simulink model "B2B_HVDC_MMC"  (R2023b)
settings: Solver=ode23t  StartTime=0.0  StopTime=3  FixedStep=Ts_Power  MaxStep=1e-3  MinStep=Ts_Power  RelTol=1e-3
values from neighbouring files (symbols this model uses):
  AC_lim = 1*[1.5 -1.5]    [B2B_HVDC_MMC_Calc.m]
  C_pm = 10.48e-3    (= 0.01048)    [B2B_HVDC_MMC_Calc.m]
  Carm = 1.0*C_pm/n    (= 0.0002096)    [B2B_HVDC_MMC_Calc.m]    (also in HVDC_MMC_param.m = 4.88333333333e-05)
  ccsc_lim = 1*[1.0 -1.0]    [B2B_HVDC_MMC_Calc.m]
  DC_lim = 1*[1.05 -1.05]    [B2B_HVDC_MMC_Calc.m]
  f = 50    [B2B_HVDC_MMC_Calc.m]
  Fn_filter = 1000    [B2B_HVDC_MMC_Calc.m]    (also in HVDC_MMC_param.m)
  Fnom = 50    [HVDC_MMC_param.m]
  HrmOrd = N    (= 2)    [B2B_HVDC_MMC_Calc.m]    (also in HVDC_MMC_param.m)
  I_nom = S_nom/(sqrt(3)*V_grid)    [B2B_HVDC_MMC_Calc.m]
  Ireg_lim_i = 1*[1.5, -1.5]    [B2B_HVDC_MMC_Calc.m]
  Ireg_lim_r = 2*[1.5, -1.5]    [B2B_HVDC_MMC_Calc.m]
  Ki_ACreg_i = 260    [B2B_HVDC_MMC_Calc.m]
  Ki_ccsc = 5    [B2B_HVDC_MMC_Calc.m]
  Ki_DCreg_r = 150    [B2B_HVDC_MMC_Calc.m]
  Ki_Ireg_i = 200    [B2B_HVDC_MMC_Calc.m]
  Ki_Ireg_r = 50    [B2B_HVDC_MMC_Calc.m]
  Kp_ACreg_i = 2    [B2B_HVDC_MMC_Calc.m]
  Kp_ccsc = 1    [B2B_HVDC_MMC_Calc.m]
  Kp_DCreg_r = 8    [B2B_HVDC_MMC_Calc.m]
  Kp_Ireg_i = 2    [B2B_HVDC_MMC_Calc.m]
  Kp_Ireg_r = 0.8    [B2B_HVDC_MMC_Calc.m]
  L1_si = L1_pu*Z_base66/w    [B2B_HVDC_MMC_Calc.m]
  L_arm = L_arm_pu*Z_base66/w    [B2B_HVDC_MMC_Calc.m]
  L_arm_pu = 0.15    [B2B_HVDC_MMC_Calc.m]
  N = 2    [B2B_HVDC_MMC_Calc.m]
  P_nom = 220e6    (= 220000000)    [B2B_HVDC_MMC_Calc.m]
  R1_si = R1_pu*Z_base66    [B2B_HVDC_MMC_Calc.m]
  R_arm = 0.03    [B2B_HVDC_MMC_Calc.m]
  R_arm_pu = R_arm/Z_base66    [B2B_HVDC_MMC_Calc.m]
  R_load = 0.6*40    (= 24)    [B2B_HVDC_MMC_Calc.m]
  R_startup = 17    [B2B_HVDC_MMC_Calc.m]    (also in HVDC_MMC_param.m = 400)
  T_fault = 1.4    [B2B_HVDC_MMC_Calc.m]
  Ts = Ts_Power    (= 5e-05)    [B2B_HVDC_MMC_Calc.m]    (also in HVDC_MMC_param.m)
  Ts_Control = Ts_Power    (= 5e-05)    [B2B_HVDC_MMC_Calc.m]    (also in HVDC_MMC_param.m)
  Ts_DQN = MultTs*Ts_Power    (= 5e-05)    [B2B_HVDC_MMC_Calc.m]    (also in HVDC_MMC_param.m)
  Ts_Power = 1*50e-6    (= 5e-05)    [B2B_HVDC_MMC_Calc.m]    (also in HVDC_MMC_param.m)
  V_ac_ref = 1.035    [B2B_HVDC_MMC_Calc.m]
  V_grid = 66e3    (= 66000)    [B2B_HVDC_MMC_Calc.m]
  Vdc_nom = 135e3    (= 135000)    [B2B_HVDC_MMC_Calc.m]
  Vnom_prim = 333e3    (= 333000)    [HVDC_MMC_param.m]
  Xdcpnz = [zeros(6,1), Xpnz]    [B2B_HVDC_MMC_Calc.m]
  Zeta_filter = 1    [B2B_HVDC_MMC_Calc.m]    (also in HVDC_MMC_param.m)
undefined symbols (not defined in the file or in its folder): DiscIntNeverNeededParam, Pcc, Xdcpnz_c
libraries: DQN_Lib x39, simulink x26, eeTransforms x21, spsCurrentMeasurementLib x16, spsHalfBridgeMMCLib x12, spsSeriesRLCBranchLib x12, B2B_HVDC_MMC_Lib x8, spsSecondOrderFilterLib x8, spsAlphaBetaZerotodq0Lib x6, spsabctoAlphaBetaZeroLib x6, spsThreePhaseVIMeasurementLib x4, spsabctodq0Lib x3
(part 1 of 5)
settings Model: NumberOfSteps=1000  SnapshotBufferSize=5000  SnapshotInterval=100  Creator=tslettba  LastModifiedBy=rober
settings SolverCC: ZeroCrossControl=DisableAll  AlgebraicLoopSolver=TrustRegion  InsertRTBMode=Never (minimum delay)  DecoupledContinuousIntegration=on  ODENIntegrationMethod=ode4
settings DataIOCC: InitialState=xFinal  SaveOperatingPoint=on  SaveFormat=Array  SaveOutput=off  SignalLogging=off  DSMLogging=off  SaveTime=off  ReturnWorkspaceOutputs=off
settings OptimizationCC: BooleanDataType=off  EfficientMapNaN2IntZero=off
settings DebuggingCC: ArithmeticOperatorsInVariantConditions=warning
settings HardwareCC: TargetBitPerPointer=64  TargetBitPerSizeT=64  TargetBitPerPtrDiffT=64  TargetLongLongMode=on  TargetIntDivRoundTo=Zero  TargetEndianess=LittleEndian  TargetWordSize=64  TargetHWDeviceType=MATLAB Host  ProdEqTarget=off
settings ModelReferenceCC: EnableRefExpFcnMdlSchedulingChecks=on  ModelReferenceMinAlgLoopOccurrences=on
settings SFSimCC: SimUseLocalCustomCode=off  CustomCodeUndefinedFunction=UseInterfaceOnly
settings RTWCC: RTWUseLocalCustomCode=off  DLArmComputeVersion=19.05
settings CodeAppCC: MaxIdLength=128
settings GRTTargetCC: TargetLangStandard=C89/C90 (ANSI)  CombineOutputUpdateFcns=off  GRTInterface=on
settings SimscapeCC: SimscapeNormalizeSystem=off

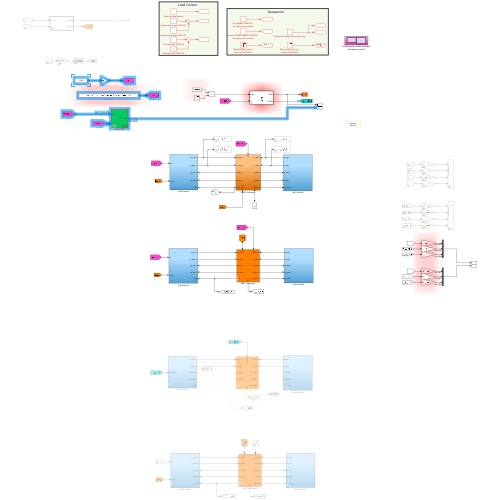
[thumbnail: Simulink's stored preview of the top-level diagram]
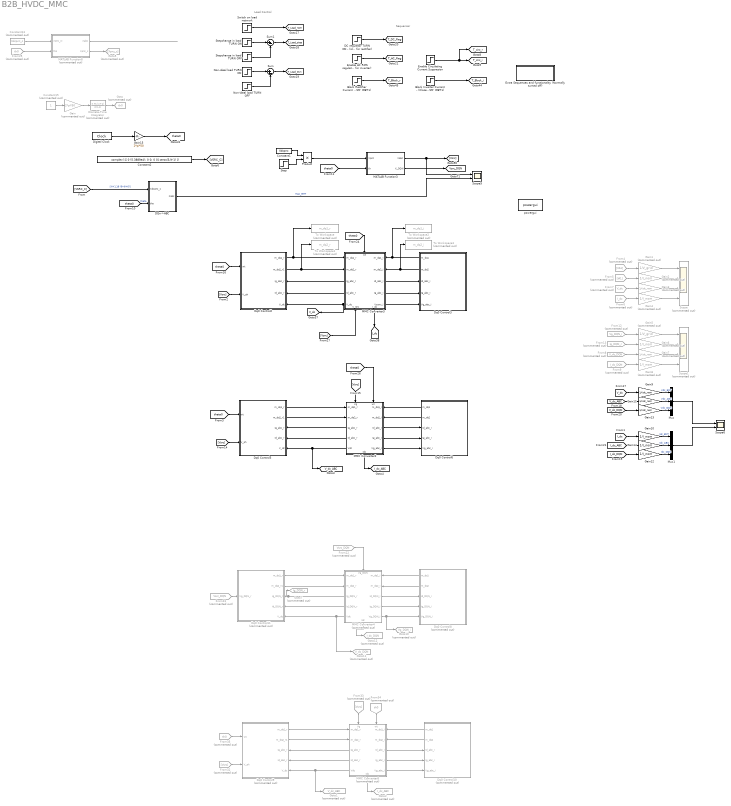
== system B2B_HVDC_MMC ==
  note: Sequencer
  note: Load Control
  Block Inverter Current - (Close all SM' IGBT's) : Step  Time=999999  SampleTime=0
  Block Rectifier Current - (Close all SM' IGBT's) : Step  Time=9999  SampleTime=0
  Constant1 : Constant  Value=Xdcpnz
  Constant13 : Constant  Commented=on  Value=Xdcpnz_c
  Constant15 : Constant  Commented=on
  Constant2 : Constant  Value=complex( [[ 0 (5.3889e4); 0 0; 0 0] zeros(3,N-1) ])
  DC regulator TURN ON - (id reference for rectifier) : Step  Time=0.4  SampleTime=0
  DQn->ABC : MATLAB Function  TreatAsAtomicUnit=on  SystemSampleTime=Ts  mask{N=N}
      mask prompts: N "Harmonic order:"
  Digital Clock : DigitalClock  SampleTime=Ts_Power
  Discrete-Time Integrator : DiscreteIntegrator  Commented=on  IntegratorMethod=Integration: Trapezoidal  SampleTime=Ts_Power  ICPrevOutput=DiscIntNeverNeededParam  ICPrevScaledInput=DiscIntNeverNeededParam
  Dq0 Control10 : Subsystem  Commented=on  VariantControl=Variant1
      settings: PortSchema="{\"entries\":[{\"content\":{\"sides\":[{\"content\":{\"connectorIds\":[]},\"type\":\"ConnectorPlacement.EquallySpacedRectSide\",\"uuid\":\"36f76858-f5b3-4aec-a766-59dc31be5bec\"},{\"content\":{\"connectorIds\":[\"Out1\",\"Out2\",\"In1\",\"In2\",\"In3\"],\"side\":\"RIGHT\"},\"type\":\"ConnectorPlacement.EquallySpacedRectSide\",\"uuid\":\"04787d34-b47d-4ffd-86c1-f3c2e1139151\"},{\"content\":{\"connectorIds\":[],\"side\":\"TOP\"},\"type\":\"ConnectorPlacement.EquallySpacedRectSide\",\"uuid\":\"4aac8492-fb89-4481-9d84-015c15a3650f\"}]},\"type\":\"ConnectorPlacement.EquallySpacedConnector\",\"uuid\":\"f0857c10-9101-4944-b9c2-34b9561f63da\"}],\"packageUris\":[\"http://schema.mathworks.com/mf0/Connector/R2020b\"],\"version\":\"1.0\"}"
  Dq0 Control11 : Subsystem  Commented=on  VariantControl=Variant1
      settings: PortSchema="{\"entries\":[{\"content\":{\"sides\":[{\"content\":{\"connectorIds\":[\"In1\"]},\"type\":\"ConnectorPlacement.EquallySpacedRectSide\",\"uuid\":\"5054124d-5268-420b-bfb4-2e4b28f216ef\"},{\"content\":{\"connectorIds\":[\"Out1\",\"Out2\",\"In2\",\"In3\",\"In4\"],\"side\":\"RIGHT\"},\"type\":\"ConnectorPlacement.EquallySpacedRectSide\",\"uuid\":\"36fdee57-87fd-4c50-8645-9d62359766d9\"},{\"content\":{\"connectorIds\":[],\"side\":\"TOP\"},\"type\":\"ConnectorPlacement.EquallySpacedRectSide\",\"uuid\":\"7247bb4b-18a5-4014-81f5-18aef71126d1\"}]},\"type\":\"ConnectorPlacement.EquallySpacedConnector\",\"uuid\":\"c58730e1-91aa-4896-a8ed-35fe7a3c59a5\"}],\"packageUris\":[\"http://schema.mathworks.com/mf0/Connector/R2020b\"],\"version\":\"1.0\"}"
  Dq0 Control2 : Subsystem  VariantControl=Variant1
      settings: PortSchema="{\"entries\":[{\"content\":{\"sides\":[{\"content\":{\"connectorIds\":[\"In1\",\"In2\"]},\"type\":\"ConnectorPlacement.EquallySpacedRectSide\",\"uuid\":\"5054124d-5268-420b-bfb4-2e4b28f216ef\"},{\"content\":{\"connectorIds\":[\"Out1\",\"Out2\",\"In3\",\"In4\",\"In5\"],\"side\":\"RIGHT\"},\"type\":\"ConnectorPlacement.EquallySpacedRectSide\",\"uuid\":\"36fdee57-87fd-4c50-8645-9d62359766d9\"},{\"content\":{\"connectorIds\":[],\"side\":\"TOP\"},\"type\":\"ConnectorPlacement.EquallySpacedRectSide\",\"uuid\":\"7247bb4b-18a5-4014-81f5-18aef71126d1\"}]},\"type\":\"ConnectorPlacement.EquallySpacedConnector\",\"uuid\":\"c58730e1-91aa-4896-a8ed-35fe7a3c59a5\"}],\"packageUris\":[\"http://schema.mathworks.com/mf0/Connector/R2020b\"],\"version\":\"1.0\"}"
  Dq0 Control3 : Subsystem  VariantControl=Variant1
      settings: PortSchema="{\"entries\":[{\"content\":{\"sides\":[{\"content\":{\"connectorIds\":[]},\"type\":\"ConnectorPlacement.EquallySpacedRectSide\",\"uuid\":\"36f76858-f5b3-4aec-a766-59dc31be5bec\"},{\"content\":{\"connectorIds\":[\"Out1\",\"Out2\",\"In1\",\"In2\",\"In3\"],\"side\":\"RIGHT\"},\"type\":\"ConnectorPlacement.EquallySpacedRectSide\",\"uuid\":\"04787d34-b47d-4ffd-86c1-f3c2e1139151\"},{\"content\":{\"connectorIds\":[],\"side\":\"TOP\"},\"type\":\"ConnectorPlacement.EquallySpacedRectSide\",\"uuid\":\"4aac8492-fb89-4481-9d84-015c15a3650f\"}]},\"type\":\"ConnectorPlacement.EquallySpacedConnector\",\"uuid\":\"f0857c10-9101-4944-b9c2-34b9561f63da\"}],\"packageUris\":[\"http://schema.mathworks.com/mf0/Connector/R2020b\"],\"version\":\"1.0\"}"
  Dq0 Control5 : Subsystem  VariantControl=Variant1
      settings: PortSchema="{\"entries\":[{\"content\":{\"sides\":[{\"content\":{\"connectorIds\":[\"In1\",\"In2\"]},\"type\":\"ConnectorPlacement.EquallySpacedRectSide\",\"uuid\":\"5054124d-5268-420b-bfb4-2e4b28f216ef\"},{\"content\":{\"connectorIds\":[\"Out1\",\"Out2\",\"In3\",\"In4\",\"In5\"],\"side\":\"RIGHT\"},\"type\":\"ConnectorPlacement.EquallySpacedRectSide\",\"uuid\":\"36fdee57-87fd-4c50-8645-9d62359766d9\"},{\"content\":{\"connectorIds\":[],\"side\":\"TOP\"},\"type\":\"ConnectorPlacement.EquallySpacedRectSide\",\"uuid\":\"7247bb4b-18a5-4014-81f5-18aef71126d1\"}]},\"type\":\"ConnectorPlacement.EquallySpacedConnector\",\"uuid\":\"c58730e1-91aa-4896-a8ed-35fe7a3c59a5\"}],\"packageUris\":[\"http://schema.mathworks.com/mf0/Connector/R2020b\"],\"version\":\"1.0\"}"
  Dq0 Control6 : Subsystem  VariantControl=Variant1
      settings: PortSchema="{\"entries\":[{\"content\":{\"sides\":[{\"content\":{\"connectorIds\":[]},\"type\":\"ConnectorPlacement.EquallySpacedRectSide\",\"uuid\":\"36f76858-f5b3-4aec-a766-59dc31be5bec\"},{\"content\":{\"connectorIds\":[\"Out1\",\"Out2\",\"In1\",\"In2\",\"In3\"],\"side\":\"RIGHT\"},\"type\":\"ConnectorPlacement.EquallySpacedRectSide\",\"uuid\":\"04787d34-b47d-4ffd-86c1-f3c2e1139151\"},{\"content\":{\"connectorIds\":[],\"side\":\"TOP\"},\"type\":\"ConnectorPlacement.EquallySpacedRectSide\",\"uuid\":\"4aac8492-fb89-4481-9d84-015c15a3650f\"}]},\"type\":\"ConnectorPlacement.EquallySpacedConnector\",\"uuid\":\"f0857c10-9101-4944-b9c2-34b9561f63da\"}],\"packageUris\":[\"http://schema.mathworks.com/mf0/Connector/R2020b\"],\"version\":\"1.0\"}"
  Dq0 Control8 : Subsystem  Commented=on  VariantControl=Variant1
      settings: PortSchema="{\"entries\":[{\"content\":{\"sides\":[{\"content\":{\"connectorIds\":[]},\"type\":\"ConnectorPlacement.EquallySpacedRectSide\",\"uuid\":\"36f76858-f5b3-4aec-a766-59dc31be5bec\"},{\"content\":{\"connectorIds\":[\"Out1\",\"Out2\",\"In1\",\"In2\",\"In3\"],\"side\":\"RIGHT\"},\"type\":\"ConnectorPlacement.EquallySpacedRectSide\",\"uuid\":\"04787d34-b47d-4ffd-86c1-f3c2e1139151\"},{\"content\":{\"connectorIds\":[],\"side\":\"TOP\"},\"type\":\"ConnectorPlacement.EquallySpacedRectSide\",\"uuid\":\"4aac8492-fb89-4481-9d84-015c15a3650f\"}]},\"type\":\"ConnectorPlacement.EquallySpacedConnector\",\"uuid\":\"f0857c10-9101-4944-b9c2-34b9561f63da\"}],\"packageUris\":[\"http://schema.mathworks.com/mf0/Connector/R2020b\"],\"version\":\"1.0\"}"
  Dq0 Control9 : Subsystem  Commented=on  VariantControl=Variant1
      settings: PortSchema="{\"entries\":[{\"content\":{\"sides\":[{\"content\":{\"connectorIds\":[\"In1\",\"In2\"]},\"type\":\"ConnectorPlacement.EquallySpacedRectSide\",\"uuid\":\"5054124d-5268-420b-bfb4-2e4b28f216ef\"},{\"content\":{\"connectorIds\":[\"Out1\",\"Out2\",\"In3\",\"In4\",\"In5\"],\"side\":\"RIGHT\"},\"type\":\"ConnectorPlacement.EquallySpacedRectSide\",\"uuid\":\"36fdee57-87fd-4c50-8645-9d62359766d9\"},{\"content\":{\"connectorIds\":[],\"side\":\"TOP\"},\"type\":\"ConnectorPlacement.EquallySpacedRectSide\",\"uuid\":\"7247bb4b-18a5-4014-81f5-18aef71126d1\"}]},\"type\":\"ConnectorPlacement.EquallySpacedConnector\",\"uuid\":\"c58730e1-91aa-4896-a8ed-35fe7a3c59a5\"}],\"packageUris\":[\"http://schema.mathworks.com/mf0/Connector/R2020b\"],\"version\":\"1.0\"}"
  Enable AC RMS regulator TURN ON - (id reference for inverter) : Step  Time=0.5  SampleTime=0  ZeroCross=off
  Enable Circulating Current Suppresion : Step  SampleTime=0
  Extra Sequences and functionality (Normally turned off) : Subsystem
  From12 : From  Commented=on  GotoTag=Vg_DQN_i  TagVisibility=global
  From13 : From  Commented=on  GotoTag=Ig_DQN_r  TagVisibility=global
  From22 : From  Commented=on  GotoTag=Vsrc_DQN  TagVisibility=global
  From23 : From  Commented=on  GotoTag=Vsrc_DQN  TagVisibility=global
  From25 : From  Commented=on  GotoTag=th0  TagVisibility=global
  From32 : From  Commented=on  GotoTag=Vsrc
  From33 : From  Commented=on  GotoTag=Vsrc
  From34 : From  Commented=on  GotoTag=th0  TagVisibility=global
  From35 : From  Commented=on  GotoTag=th0  TagVisibility=global
  From4 : From  Commented=on  GotoTag=VA1  TagVisibility=global
  From5 : From  Commented=on  GotoTag=IA1  TagVisibility=global
  From6 : From  Commented=on  GotoTag=I_dc  TagVisibility=global
  From7 : From  Commented=on  GotoTag=V_dc  TagVisibility=global
  From8 : From  Commented=on  GotoTag=V_dc_DQN  TagVisibility=global
  From9 : From  Commented=on  GotoTag=I_dc_DQN  TagVisibility=global
  Gain : Gain  Commented=on  Gain=2*pi*50
  Gain1 : Gain  Commented=on  Gain=1/V_grid
  Gain10 : Gain  Gain=1/I_nom
  Gain11 : Gain  Gain=1/Vdc_nom
  Gain12 : Gain  Gain=1/I_nom
  Gain13 : Gain  Gain=1/Vdc_nom
  Gain14 : Gain  Gain=1/I_nom
  Gain15 : Gain  Gain=2*pi*50
  Gain{2,4,6,8} (4 alike) : Gain  Commented=on  Gain=1/I_nom
  Gain3 : Gain  Commented=on  Gain=1/Vdc_nom
  Gain5 : Gain  Commented=on  Gain=1/V_grid
  Gain7 : Gain  Commented=on  Gain=1/Vdc_nom
  Gain9 : Gain  Gain=1/Vdc_nom
  Goto : Goto  Commented=on  GotoTag=th0  TagVisibility=global
  Goto1 : Goto  Commented=on  GotoTag=V_dc_ABC  TagVisibility=global
  Goto10 : Goto  Commented=on  GotoTag=Vg_DQN_i  TagVisibility=global
  Goto11 : Goto  Commented=on  GotoTag=V_dc_DQN  TagVisibility=global
  Goto12 : Goto  Commented=on  GotoTag=I_dc_DQN  TagVisibility=global
  Goto2 : Goto  Commented=on  GotoTag=I_dc_ABC  TagVisibility=global
  Goto5 : Goto  Commented=on  GotoTag=Xpnz_c
  Goto7 : Goto  Commented=on  GotoTag=Ig_DQN_r  TagVisibility=global
  MATLAB Function3 : MATLAB Function  TreatAsAtomicUnit=on  mask{chkHrmLst=off, HRM=N, HrmLst=[0 7 8]}
      mask prompts: chkHrmLst "Only specific harmonics"; HRM "Harmonic order:"; HrmLst "Harmonic list:"
  MATLAB Function8 : MATLAB Function  Commented=on  TreatAsAtomicUnit=on  mask{chkHrmLst=off, HRM=N, HrmLst=[0 7 8]}
      mask prompts: chkHrmLst "Only specific harmonics"; HRM "Harmonic order:"; HrmLst "Harmonic list:"
  MMC Converter2 : Subsystem  mask{Ts_Power=Ts_DQN}
      mask prompts: Ts_Power "Sample time:"
      settings: PortSchema="{\"entries\":[{\"content\":{\"sides\":[{\"content\":{\"connectorIds\":[\"In1\",\"In2\",\"Out5\",\"Out6\",\"Out7\"]},\"type\":\"ConnectorPlacement.EquallySpacedRectSide\",\"uuid\":\"87652525-d4f3-48bd-afb9-55813d4b97b9\"},{\"content\":{\"connectorIds\":[\"In5\",\"In6\",\"Out1\",\"Out2\",\"Out3\"],\"side\":\"RIGHT\"},\"type\":\"ConnectorPlacement.EquallySpacedRectSide\",\"uuid\":\"55382f73-b2a1-4e3c-9356-c55b2c306da5\"},{\"content\":{\"connectorIds\":[\"In3\",\"In4\"],\"side\":\"TOP\"},\"type\":\"ConnectorPlacement.EquallySpacedRectSide\",\"uuid\":\"5746e390-86c5-411c-b1f1-99edaaeabbe1\"},{\"content\":{\"connectorIds\":[\"Out4\"],\"side\":\"BOTTOM\"},\"type\":\"ConnectorPlacement.EquallySpacedRectSide\",\"uuid\":\"499a406e-551e-409c-998b-1d8f3bc160f4\"}]},\"type\":\"ConnectorPlacement.EquallySpacedConnector\",\"uuid\":\"6141d85e-66b3-4906-aa89-7ac82b0805e9\"}],\"packageUris\":[\"http://schema.mathworks.com/mf0/Connector/R2020b\"],\"version\":\"1.0\"}"
  MMC Converter3 : Subsystem
      settings: PortSchema="{\"entries\":[{\"content\":{\"sides\":[{\"content\":{\"connectorIds\":[\"In1\",\"In2\",\"Out5\",\"Out6\",\"Out7\"]},\"type\":\"ConnectorPlacement.EquallySpacedRectSide\",\"uuid\":\"87652525-d4f3-48bd-afb9-55813d4b97b9\"},{\"content\":{\"connectorIds\":[\"In5\",\"In6\",\"Out1\",\"Out2\",\"Out3\"],\"side\":\"RIGHT\"},\"type\":\"ConnectorPlacement.EquallySpacedRectSide\",\"uuid\":\"55382f73-b2a1-4e3c-9356-c55b2c306da5\"},{\"content\":{\"connectorIds\":[\"In3\"],\"side\":\"TOP\"},\"type\":\"ConnectorPlacement.EquallySpacedRectSide\",\"uuid\":\"5746e390-86c5-411c-b1f1-99edaaeabbe1\"},{\"content\":{\"connectorIds\":[\"In4\",\"Out4\"],\"side\":\"BOTTOM\"},\"type\":\"ConnectorPlacement.EquallySpacedRectSide\",\"uuid\":\"499a406e-551e-409c-998b-1d8f3bc160f4\"}]},\"type\":\"ConnectorPlacement.EquallySpacedConnector\",\"uuid\":\"6141d85e-66b3-4906-aa89-7ac82b0805e9\"}],\"packageUris\":[\"http://schema.mathworks.com/mf0/Connector/R2020b\"],\"version\":\"1.0\"}"
  MMC Converter4 : Subsystem  Commented=on  mask{Ts_Power=Ts_DQN}
      mask prompts: Ts_Power "Sample time (s):"
      settings: PortSchema="{\"entries\":[{\"content\":{\"sides\":[{\"content\":{\"connectorIds\":[\"In1\",\"In2\",\"Out5\",\"Out6\",\"Out7\"]},\"type\":\"ConnectorPlacement.EquallySpacedRectSide\",\"uuid\":\"87652525-d4f3-48bd-afb9-55813d4b97b9\"},{\"content\":{\"connectorIds\":[\"In4\",\"In5\",\"Out1\",\"Out2\",\"Out3\"],\"side\":\"RIGHT\"},\"type\":\"ConnectorPlacement.EquallySpacedRectSide\",\"uuid\":\"55382f73-b2a1-4e3c-9356-c55b2c306da5\"},{\"content\":{\"connectorIds\":[\"In3\"],\"side\":\"TOP\"},\"type\":\"ConnectorPlacement.EquallySpacedRectSide\",\"uuid\":\"5746e390-86c5-411c-b1f1-99edaaeabbe1\"},{\"content\":{\"connectorIds\":[\"Out4\"],\"side\":\"BOTTOM\"},\"type\":\"ConnectorPlacement.EquallySpacedRectSide\",\"uuid\":\"499a406e-551e-409c-998b-1d8f3bc160f4\"}]},\"type\":\"ConnectorPlacement.EquallySpacedConnector\",\"uuid\":\"6141d85e-66b3-4906-aa89-7ac82b0805e9\"}],\"packageUris\":[\"http://schema.mathworks.com/mf0/Connector/R2020b\"],\"version\":\"1.0\"}"
  MMC Converter8 : Subsystem  Commented=on  mask{Ts_Power=Ts_DQN}
      mask prompts: Ts_Power "Sample time:"
      settings: PortSchema="{\"entries\":[{\"content\":{\"sides\":[{\"content\":{\"connectorIds\":[\"In1\",\"In2\",\"Out5\",\"Out6\",\"Out7\"]},\"type\":\"ConnectorPlacement.EquallySpacedRectSide\",\"uuid\":\"87652525-d4f3-48bd-afb9-55813d4b97b9\"},{\"content\":{\"connectorIds\":[\"In5\",\"In6\",\"Out1\",\"Out2\",\"Out3\"],\"side\":\"RIGHT\"},\"type\":\"ConnectorPlacement.EquallySpacedRectSide\",\"uuid\":\"55382f73-b2a1-4e3c-9356-c55b2c306da5\"},{\"content\":{\"connectorIds\":[\"In3\",\"In4\"],\"side\":\"TOP\"},\"type\":\"ConnectorPlacement.EquallySpacedRectSide\",\"uuid\":\"5746e390-86c5-411c-b1f1-99edaaeabbe1\"},{\"content\":{\"connectorIds\":[\"Out4\"],\"side\":\"BOTTOM\"},\"type\":\"ConnectorPlacement.EquallySpacedRectSide\",\"uuid\":\"499a406e-551e-409c-998b-1d8f3bc160f4\"}]},\"type\":\"ConnectorPlacement.EquallySpacedConnector\",\"uuid\":\"6141d85e-66b3-4906-aa89-7ac82b0805e9\"}],\"packageUris\":[\"http://schema.mathworks.com/mf0/Connector/R2020b\"],\"version\":\"1.0\"}"
  Mux : Mux  Inputs=3
  Mux1 : Mux  Inputs=3
  Non-ideal load TURN OFF : Step  Time=2.2*999  SampleTime=0
  Non-ideal load TURN ON : Step  Time=0.7  SampleTime=0
  Product : Product
  Scope : Scope  Commented=on  NumInputPorts=4
  Scope1 : Scope  Commented=on  NumInputPorts=4
  Scope5 : Scope  NumInputPorts=2
  Scope6 : Scope  NumInputPorts=2
  Step : Step  Time=2  Before=1  After=1.15  SampleTime=0
  Stepchange in load TURN OFF : Step  Time=999  SampleTime=0
  Stepchange in load TURN ON : Step  Time=2*9999999  SampleTime=0
  Sum : Sum  Inputs=|+-
  Sum1 : Sum  Inputs=|+-
  Switch on load network : Step  Time=0.3+0*0.6  SampleTime=0
  To Workspace : ToWorkspace  Commented=on  VariableName=m_dq1_r  SaveFormat=Timeseries  SampleTime=Ts_Power
      settings: MaxDataPoints=1
  To Workspace1 : ToWorkspace  Commented=on  VariableName=m_dq2_r  SaveFormat=Timeseries  SampleTime=Ts_Power
      settings: MaxDataPoints=1
  To Workspace2 : ToWorkspace  Commented=on  VariableName=m_dq1_i  SaveFormat=Timeseries  SampleTime=Ts_Power
      settings: MaxDataPoints=1
  To Workspace3 : ToWorkspace  Commented=on  VariableName=m_dq2_i  SaveFormat=Timeseries  SampleTime=Ts_Power
      settings: MaxDataPoints=1
  powergui : spspowerguiLib/powergui  Priority=1  SimulationMode=Discrete  SampleTime=Ts_Power  frequency=60  Iterations=50  frequencyindice=50  Pbase=100e6  ErrMax=1e-4  UnitsV=kV  UnitsW=MW  buscounter=0  FunctionMessages=off  echomessages=off  EnableUseOfTLC=off  CurrentSourceSwitches=off  DisableSnubberDevices=off  DisableRonSwitches=off  DisableVfSwitches=off  DisplayEquations=off  AutomaticDiscreteSolvers=on  SolverType=Tustin/Backward Euler (TBE)  Interpol=off  ExternalGateDelay=off  methode=off  Ts=100  x0status=blocks  SPID=on  SwTol=0  HookPort=off  NonlinearTolerance=1e-4  nMaxIteration=100  ContinueOnMaxIteration=off  RestoreLinks=warning  ResistiveCurrentMeasurement=off  Frange=[0:10:1000000]  Ylog=off  Xlog=on  ShowGrid=on  save=off  variable=ZData  structure=I_inv  ZoomFFT=off  StartTime=2  cycles=1  DisplayStyle=1  fundamental=50  FreqAxis=on  MaxFrequency=3000  frequencyindicesteady=1  RmsSteady=1  display=off
  tag scope: I_dc=global, I_dc_ABC=global, T_AC_Reg=global, T_Block_i=global, T_Block_r=global, T_DC_Reg=global, T_Load_Dyn=global, T_Load_nom=global, T_Load_step=global, T_circ_i=global, T_circ_r=global, V_dc=global, V_dc_ABC=global, Vsrc_DQN=global, theta0=global
  wires:
  Non-ideal load TURN ON/1 -> Sum/1
  Non-ideal load TURN OFF/1 -> Sum/2
  Switch on load network/1 -> [T_Load_nom]
  Sum/1 -> [T_Load_Dyn]
  Stepchange in load TURN OFF/1 -> Sum1/2
  Stepchange in load TURN ON/1 -> Sum1/1
  Sum1/1 -> [T_Load_step]
  DC regulator TURN ON - (id reference for rectifier)/1 -> [T_DC_Reg]
  Enable AC RMS regulator TURN ON - (id reference for inverter)/1 -> [T_AC_Reg]
  Enable Circulating Current Suppresion/1 -> [T_circ_r], [T_circ_i]
  Block Inverter Current - (Close all SM' IGBT's)/1 -> [T_Block_i]
  Block Rectifier Current - (Close all SM' IGBT's)/1 -> [T_Block_r]
  Constant15/1 -> Gain/1
  Discrete-Time Integrator/1 -> Goto/1
  Gain/1 -> Discrete-Time Integrator/1
  MMC Converter3/2(Ig_abc_i) -> Dq0 Control3/2(Ig_abc_i)
  Dq0 Control2/2(m_dq2_r1) -> To Workspace1/1, MMC Converter3/2(m_dq2_r)
  Dq0 Control3/1(m_dq1) -> To Workspace2/1, MMC Converter3/5(m_dq1_i)
  MMC Converter3/6(Id_abc_r) -> Dq0 Control2/4(Id_abc_r)
  MMC Converter3/7(V_dc) -> Dq0 Control2/5(V_dc), [V_dc]
  MMC Converter3/1(Id_abc_i) -> Dq0 Control3/1(Id_abc_i)
  Dq0 Control3/2(m_dq2) -> To Workspace3/1, MMC Converter3/6(m_dq2_i)
  [theta0] -> MMC Converter3/3(wt)
  MMC Converter3/3(Vconv_i) -> Dq0 Control3/3(Vg_abc_i)
  Dq0 Control2/1(m_dq1_r) -> To Workspace/1, MMC Converter3/1(m_dq1_r)
  MMC Converter3/4(I_dc) -> [I_dc]
  [Vsrc] -> Dq0 Control2/2(V_ph)
  [theta0] -> Dq0 Control2/1(wt)
  MMC Converter3/5(Ig_abc_r) -> Dq0 Control2/3(Ig_abc_r)
  Constant1/1 -> Product/1
  Step/1 -> Product/2
  MATLAB Function3/2(X_DQN) -> [Vsrc_DQN]
  MATLAB Function3/1(Xabc) -> Scope5/1, [Vsrc]
  [theta0] -> MATLAB Function3/2(th)
  Product/1 -> MATLAB Function3/1(Xpnz)
  Gain1/1 -> Scope/1
  Gain2/1 -> Scope/2
  Gain3/1 -> Scope/3
  Gain4/1 -> Scope/4
  Gain7/1 -> Scope1/3
  Gain8/1 -> Scope1/4
  From9/1 -> Gain8/1
  From8/1 -> Gain7/1
  Gain6/1 -> Scope1/2
  From12/1 -> Gain5/1
  Gain5/1 -> Scope1/1
  From13/1 -> Gain6/1
  From5/1 -> Gain2/1
  From7/1 -> Gain3/1
  From4/1 -> Gain1/1
  From6/1 -> Gain4/1
  [Vsrc] -> MMC Converter3/4(V_Src)
  MMC Converter2/2(Ig_abc_i) -> Dq0 Control6/2(Ig_abc_i)
  [Vsrc] -> Dq0 Control5/2(V_ph)
  [theta0] -> MMC Converter2/4(wt)
  MMC Converter2/5(Ig_abc_r) -> Dq0 Control5/3(Ig_abc_r)
  [Vsrc] -> MMC Converter2/3(Vg)
  MMC Converter2/3(Vg_abc_i) -> Dq0 Control6/3(Vg_abc_i)
  MMC Converter2/1(Id_abc_i) -> Dq0 Control6/1(Id_abc_i)
  MMC Converter2/6(Id_abc_r) -> Dq0 Control5/4(Id_abc_r)
  [theta0] -> Dq0 Control5/1(wt)
  Mux1/1 -> Scope6/2
  Mux/1 -> Scope6/1
  [I_dc] -> Gain10/1
  [I_dc_DQN] -> Gain12/1
  Gain11/1 -> Mux/2  "Vdc_ABC"
  [V_dc_DQN] -> Gain13/1
  Gain13/1 -> Mux/3  "Vdc_DQN"
  [V_dc] -> Gain9/1
  [V_dc_ABC] -> Gain11/1
  Gain9/1 -> Mux/1  "Vdc_EMT"
  Gain10/1 -> Mux1/1  "Idc_EMT"
  Gain12/1 -> Mux1/3  "Idc_DQN"
  [I_dc_ABC] -> Gain14/1
  Gain14/1 -> Mux1/2  "Idc_ABC"
  Dq0 Control11/2(m_dq2_r1) -> MMC Converter4/2(m_dq2_r)
  From22/1 -> MMC Converter4/3(Vg_DQN)
  Dq0 Control8/1(m_dq1) -> MMC Converter4/4(m_dq1_i)
  Dq0 Control11/1(m_dq1_r) -> MMC Converter4/1(m_dq1_r)
  Dq0 Control8/2(m_dq2) -> MMC Converter4/5(m_dq2_i)
  From23/1 -> Dq0 Control11/1(Vg_DQN_r)
  MMC Converter4/4(Idc) -> Goto12/1
  MMC Converter4/5(Ig_DQN_r) -> Goto7/1, Dq0 Control11/2(Ig_DQN_r)
  MMC Converter4/6(Id_DQN_r) -> Dq0 Control11/3(Id_DQN_r)
  MMC Converter4/1(Id_DQN_i) -> Dq0 Control8/1(Id_DQN_i)
  MMC Converter4/2(Ig_DQN_i) -> Dq0 Control8/2(Ig_DQN_i)
  MMC Converter4/3(Vg_DQN_i) -> Dq0 Control8/3(Vg_DQN_i), Goto10/1
  Dq0 Control5/1(m_dq1_r) -> MMC Converter2/1(m_dq1_r)
  Dq0 Control5/2(m_dq2_r1) -> MMC Converter2/2(m_dq2_r)
  Dq0 Control6/1(m_dq1) -> MMC Converter2/5(m_dq1_i)
  Dq0 Control6/2(m_dq2) -> MMC Converter2/6(m_dq2_i)
  MMC Converter8/3(Vg_abc_i) -> Dq0 Control10/3(Vg_abc_i)
  MMC Converter8/5(Ig_abc_r) -> Dq0 Control9/3(Ig_abc_r)
  MMC Converter8/6(Id_abc_r) -> Dq0 Control9/4(Id_abc_r)
  MMC Converter8/1(Id_abc_i) -> Dq0 Control10/1(Id_abc_i)
  From34/1 -> MMC Converter8/4(wt)
  From32/1 -> Dq0 Control9/2(V_ph)
  MMC Converter8/7(Vdc) -> Dq0 Control9/5(V_dc), Goto1/1
  From35/1 -> Dq0 Control9/1(wt)
  From33/1 -> MMC Converter8/3(Vg)
  Dq0 Control10/2(m_dq2) -> MMC Converter8/6(m_dq2_i)
  MMC Converter8/4(Idc) -> Goto2/1
  Dq0 Control10/1(m_dq1) -> MMC Converter8/5(m_dq1_i)
  Dq0 Control9/1(m_dq1_r) -> MMC Converter8/1(m_dq1_r)
  MMC Converter8/2(Ig_abc_i) -> Dq0 Control10/2(Ig_abc_i)
  Dq0 Control9/2(m_dq2_r1) -> MMC Converter8/2(m_dq2_r)
  MMC Converter2/4(Idc) -> [I_dc_ABC]
  MMC Converter2/7(Vdc) -> [V_dc_ABC], Dq0 Control5/5(V_dc)
  MMC Converter4/7(Vdc) -> Dq0 Control11/4(V_dc), Goto11/1
  Gain15/1 -> [theta0]
  Digital Clock/1 -> Gain15/1
  From25/1 -> MATLAB Function8/2(tho)
  MATLAB Function8/1(Xabc) -> ?
  MATLAB Function8/2(Xpnz_c) -> Goto5/1
  Constant13/1 -> MATLAB Function8/1(Xpnz_ci)
  Constant2/1 -> [VSRC_C]
  [theta0] -> DQn->ABC/2(tho)  "theta"
  [VSRC_C] -> DQn->ABC/1(Xdcpnz_c)  "[N+1,18 (6+6+6)]"
  DQn->ABC/1(Xabc) -> Scope5/2  "Mac_EMT"

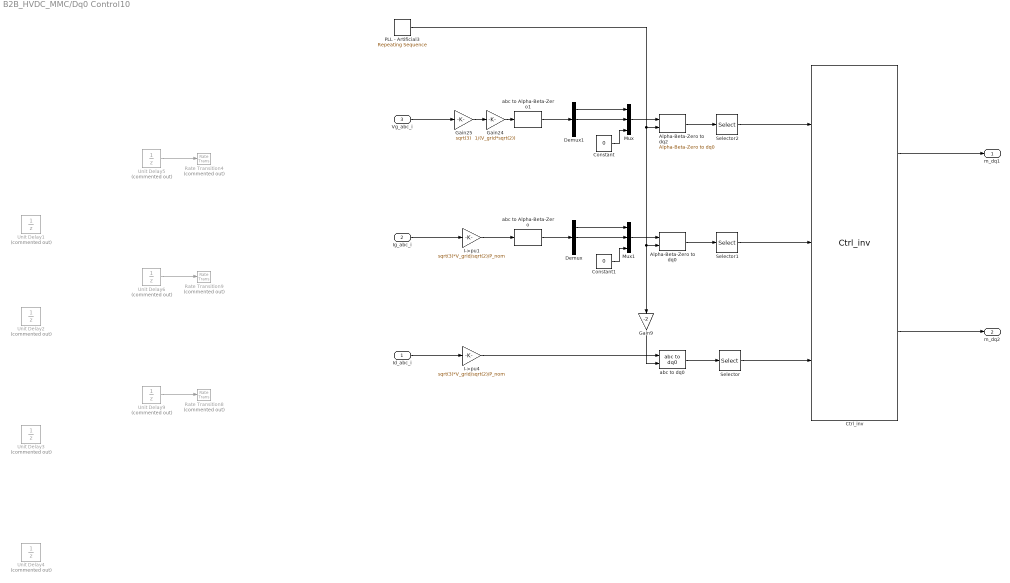
== system B2B_HVDC_MMC/Dq0 Control10 ==
  Id_abc_i : Inport
  Ig_abc_i : Inport  Port=2
  Vg_abc_i : Inport  Port=3
  Alpha-Beta-Zero to dq0 : spsAlphaBetaZerotodq0Lib/Alpha-Beta-Zero to dq0  Alignment=90 degrees behind phase A axis
  Alpha-Beta-Zero to dq2 : spsAlphaBetaZerotodq0Lib/Alpha-Beta-Zero to dq0  Alignment=90 degrees behind phase A axis
  Constant : Constant  Value=0
  Constant1 : Constant  Value=0
  Ctrl_inv : B2B_HVDC_MMC_Lib/Ctrl_inv  SystemSampleTime=-1  VariantActivationTime=update diagram  AllowFlexibleInterface=on  Latency=0  AutoFrameSizeCalculation=off
      settings: SourceProductName=BackToBack HVDC MMC Library
  Demux : Demux  Outputs=3
  Demux1 : Demux  Outputs=3
  Gain24 : Gain  Gain=1/(V_grid*sqrt(2))
  Gain25 : Gain  Gain=sqrt(3)
  Gain9 : Gain  Gain=-2
  I->pu1 : Gain  Gain=sqrt(3)*V_grid/sqrt(2)/P_nom  SaturateOnIntegerOverflow=on  OutDataTypeStr=Inherit: Same as input  ParamDataTypeStr=Inherit: Same as input
  I->pu4 : Gain  Gain=sqrt(3)*V_grid/sqrt(2)/P_nom  SaturateOnIntegerOverflow=on  OutDataTypeStr=Inherit: Same as input  ParamDataTypeStr=Inherit: Same as input
  Mux : Mux  Inputs=3
  Mux1 : Mux  Inputs=3
  PLL - Artificial3 : simulink/Sources/Repeating Sequence  rep_seq_t=[0 1/f]  rep_seq_y=[0 2*pi]
  Rate Transition4 : RateTransition  Commented=on  OutPortSampleTime=Ts_Control
  Rate Transition8 : RateTransition  Commented=on  OutPortSampleTime=Ts_Control
  Rate Transition9 : RateTransition  Commented=on  OutPortSampleTime=Ts_Control
  Selector : Selector  InputPortWidth=3  IndexOptions=Index vector (dialog)  Indices=[1 2]  OutputSizes=1
  Selector1 : Selector  InputPortWidth=3  IndexOptions=Index vector (dialog)  Indices=[1 2]  OutputSizes=1
  Selector2 : Selector  InputPortWidth=3  IndexOptions=Index vector (dialog)  Indices=[1 2]  OutputSizes=1
  Unit Delay{1..6,9} (7 alike) : UnitDelay  Commented=on  SampleTime=Ts_Power  HasFrameUpgradeWarning=on
  abc to Alpha-Beta-Zero : spsabctoAlphaBetaZeroLib/abc to Alpha-Beta-Zero
  abc to Alpha-Beta-Zero1 : spsabctoAlphaBetaZeroLib/abc to Alpha-Beta-Zero
  abc to dq0 : spsabctodq0Lib/abc to dq0  Alignment=90 degrees behind phase A axis
  m_dq1 : Outport  VectorParamsAs1DForOutWhenUnconnected=off
  m_dq2 : Outport  Port=2  VectorParamsAs1DForOutWhenUnconnected=off
  wires:
  Constant/1 -> Mux/3
  Demux/2 -> Mux1/2
  Demux/1 -> Mux1/1
  Mux1/1 -> Alpha-Beta-Zero to dq0/1
  Demux1/1 -> Mux/1
  Demux1/2 -> Mux/2
  Mux/1 -> Alpha-Beta-Zero to dq2/1
  abc to Alpha-Beta-Zero1/1 -> Demux1/1
  Alpha-Beta-Zero to dq2/1 -> Selector2/1
  Gain24/1 -> abc to Alpha-Beta-Zero1/1
  abc to Alpha-Beta-Zero/1 -> Demux/1
  I->pu1/1 -> abc to Alpha-Beta-Zero/1
  Gain25/1 -> Gain24/1
  Constant1/1 -> Mux1/3
  PLL - Artificial3/1 -> Alpha-Beta-Zero to dq2/2, Alpha-Beta-Zero to dq0/2, Gain9/1
  Gain9/1 -> abc to dq0/2
  I->pu4/1 -> abc to dq0/1
  Selector2/1 -> Ctrl_inv/1
  Selector1/1 -> Ctrl_inv/2
  Selector/1 -> Ctrl_inv/3
  Ctrl_inv/1 -> m_dq1/1
  Ctrl_inv/2 -> m_dq2/1
  Alpha-Beta-Zero to dq0/1 -> Selector1/1
  abc to dq0/1 -> Selector/1
  Unit Delay9/1 -> Rate Transition8/1
  Unit Delay6/1 -> Rate Transition9/1
  Unit Delay5/1 -> Rate Transition4/1
  Vg_abc_i/1 -> Gain25/1
  Ig_abc_i/1 -> I->pu1/1
  Id_abc_i/1 -> I->pu4/1

== system B2B_HVDC_MMC/Dq0 Control11 ==
  Vg_DQN_r : Inport
  Ig_DQN_r : Inport  Port=2
  Id_DQN_r : Inport  Port=3
  V_dc : Inport  Port=4
  Ctrl_rec : B2B_HVDC_MMC_Lib/Ctrl_rec  SystemSampleTime=-1  VariantActivationTime=update diagram  AllowFlexibleInterface=on  Latency=0  AutoFrameSizeCalculation=off
      settings: SourceProductName=BackToBack HVDC MMC Library
  Gain1 : Gain  Gain=1/(V_grid*sqrt(2))
  Gain2 : Gain  Gain=sqrt(3)
  I->pu2 : Gain  Gain=sqrt(3)*V_grid/sqrt(2)/P_nom  SaturateOnIntegerOverflow=on  OutDataTypeStr=Inherit: Same as input  ParamDataTypeStr=Inherit: Same as input
  I->pu3 : Gain  Gain=sqrt(3)*V_grid/sqrt(2)/P_nom  SaturateOnIntegerOverflow=on  OutDataTypeStr=Inherit: Same as input  ParamDataTypeStr=Inherit: Same as input
  Second-Order Filter1 : spsSecondOrderFilterLib/Second-Order Filter  FilterType=Lowpass  Fo=Fn_filter  Zeta=Zeta_filter  Ts=Ts_Control  Initialize=off  Vac_Init="[0,  0,  60]"  Vdc_Init=0  PlotResponse=off  FreqRange=[0, 500, 1]
  Selector3 : Selector  InputPortWidth=6*(N+1)  IndexOptions=Index vector (dialog)  Indices=[1*(N+1)+3 4*(N+1)+3]  OutputSizes=1
  Selector4 : Selector  InputPortWidth=6*(N+1)  IndexOptions=Index vector (dialog)  Indices=[2 3*(N+1)+2]  OutputSizes=1
  Selector5 : Selector  InputPortWidth=6*(N+1)  IndexOptions=Index vector (dialog)  Indices=[2 3*(N+1)+2]  OutputSizes=1
  Subsystem1 : Subsystem  Commented=on
  Unit Delay5 : UnitDelay  Commented=on  SampleTime=Ts_Power  HasFrameUpgradeWarning=on
  Unit Delay6 : UnitDelay  Commented=on  SampleTime=Ts_Power  HasFrameUpgradeWarning=on
  Unit Delay9 : UnitDelay  Commented=on  SampleTime=Ts_Power  HasFrameUpgradeWarning=on
  m_dq1_r : Outport
  m_dq2_r1 : Outport  Port=2
  wires:
  Selector5/1 -> Second-Order Filter1/1
  Gain1/1 -> Selector5/1
  Selector4/1 -> Ctrl_rec/2
  Selector3/1 -> Ctrl_rec/4
  V_dc/1 -> Ctrl_rec/1
  I->pu3/1 -> Selector4/1
  Gain2/1 -> Gain1/1
  I->pu2/1 -> Selector3/1
  Vg_DQN_r/1 -> Gain2/1
  Id_DQN_r/1 -> I->pu2/1
  Ig_DQN_r/1 -> I->pu3/1
  Second-Order Filter1/1 -> Ctrl_rec/3
  Ctrl_rec/1 -> m_dq1_r/1
  Ctrl_rec/2 -> m_dq2_r1/1

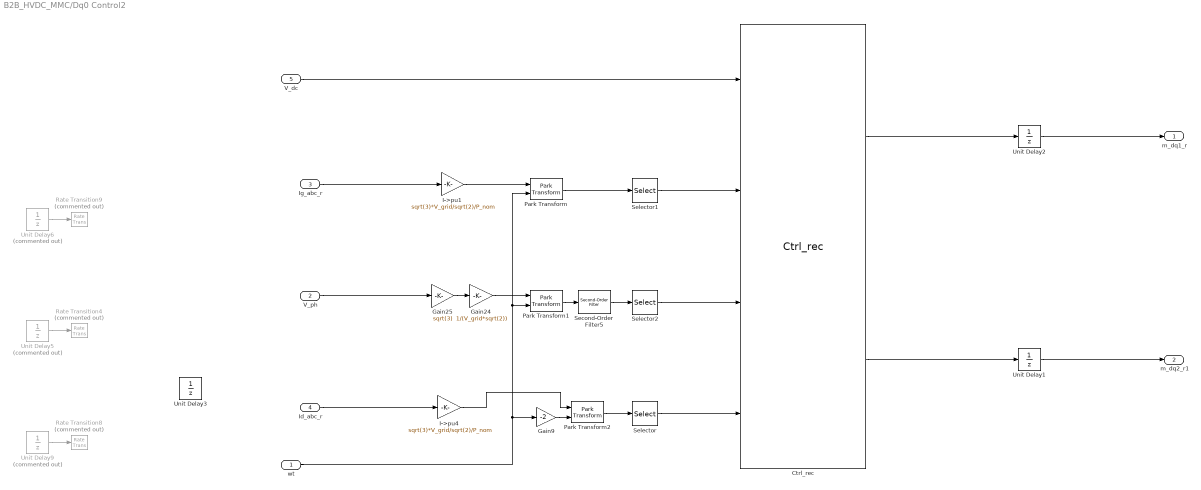
== system B2B_HVDC_MMC/Dq0 Control2 ==
  wt : Inport
  V_ph : Inport  Port=2
  Ig_abc_r : Inport  Port=3
  Id_abc_r : Inport  Port=4
  V_dc : Inport  Port=5
  Ctrl_rec : B2B_HVDC_MMC_Lib/Ctrl_rec  SystemSampleTime=-1  VariantActivationTime=update diagram  AllowFlexibleInterface=on  Latency=0  AutoFrameSizeCalculation=off
      settings: SourceProductName=BackToBack HVDC MMC Library
  Gain24 : Gain  Gain=1/(V_grid*sqrt(2))
  Gain25 : Gain  Gain=sqrt(3)
  Gain9 : Gain  Gain=-2
  I->pu1 : Gain  Gain=sqrt(3)*V_grid/sqrt(2)/P_nom  SaturateOnIntegerOverflow=on  OutDataTypeStr=Inherit: Same as input  ParamDataTypeStr=Inherit: Same as input
  I->pu4 : Gain  Gain=sqrt(3)*V_grid/sqrt(2)/P_nom  SaturateOnIntegerOverflow=on  OutDataTypeStr=Inherit: Same as input  ParamDataTypeStr=Inherit: Same as input
  Park Transform : eeTransforms/Park Transform  AxisAlignment=Q-axis  PowerInvariant=off
  Park Transform1 : eeTransforms/Park Transform  AxisAlignment=Q-axis  PowerInvariant=off
  Park Transform2 : eeTransforms/Park Transform  AxisAlignment=Q-axis  PowerInvariant=off
  Rate Transition4 : RateTransition  Commented=on  OutPortSampleTime=Ts_Control
  Rate Transition8 : RateTransition  Commented=on  OutPortSampleTime=Ts_Control
  Rate Transition9 : RateTransition  Commented=on  OutPortSampleTime=Ts_Control
  Second-Order Filter5 : spsSecondOrderFilterLib/Second-Order Filter  FilterType=Lowpass  Fo=Fn_filter  Zeta=Zeta_filter  Ts=Ts_Control  Initialize=off  Vac_Init="[0,  0,  60]"  Vdc_Init=0  PlotResponse=off  FreqRange=[0, 500, 1]
  Selector : Selector  InputPortWidth=3  IndexOptions=Index vector (dialog)  Indices=[1 2]  OutputSizes=1
  Selector1 : Selector  InputPortWidth=3  IndexOptions=Index vector (dialog)  Indices=[1 2]  OutputSizes=1
  Selector2 : Selector  InputPortWidth=3  IndexOptions=Index vector (dialog)  Indices=[1 2]  OutputSizes=1
  Unit Delay1 : UnitDelay  SampleTime=Ts_Power  HasFrameUpgradeWarning=on
  Unit Delay2 : UnitDelay  SampleTime=Ts_Power  HasFrameUpgradeWarning=on
  Unit Delay3 : UnitDelay  SampleTime=Ts_Power  HasFrameUpgradeWarning=on
  Unit Delay5 : UnitDelay  Commented=on  SampleTime=Ts_Power  HasFrameUpgradeWarning=on
  Unit Delay6 : UnitDelay  Commented=on  SampleTime=Ts_Power  HasFrameUpgradeWarning=on
  Unit Delay9 : UnitDelay  Commented=on  SampleTime=Ts_Power  HasFrameUpgradeWarning=on
  m_dq1_r : Outport
  m_dq2_r1 : Outport  Port=2
  wires:
  I->pu1/1 -> Park Transform/1
  Gain25/1 -> Gain24/1
  Second-Order Filter5/1 -> Selector2/1
  Park Transform1/1 -> Second-Order Filter5/1
  Gain24/1 -> Park Transform1/1
  wt/1 -> Gain9/1, Park Transform1/2, Park Transform/2
  Gain9/1 -> Park Transform2/2
  Park Transform2/1 -> Selector/1
  V_dc/1 -> Ctrl_rec/1
  Selector1/1 -> Ctrl_rec/2
  Selector2/1 -> Ctrl_rec/3
  Selector/1 -> Ctrl_rec/4
  Ctrl_rec/1 -> Unit Delay2/1
  Ctrl_rec/2 -> Unit Delay1/1
  I->pu4/1 -> Park Transform2/1
  Unit Delay9/1 -> Rate Transition8/1
  Unit Delay6/1 -> Rate Transition9/1
  Unit Delay5/1 -> Rate Transition4/1
  V_ph/1 -> Gain25/1
  Ig_abc_r/1 -> I->pu1/1
  Id_abc_r/1 -> I->pu4/1
  Park Transform/1 -> Selector1/1
  Unit Delay2/1 -> m_dq1_r/1
  Unit Delay1/1 -> m_dq2_r1/1

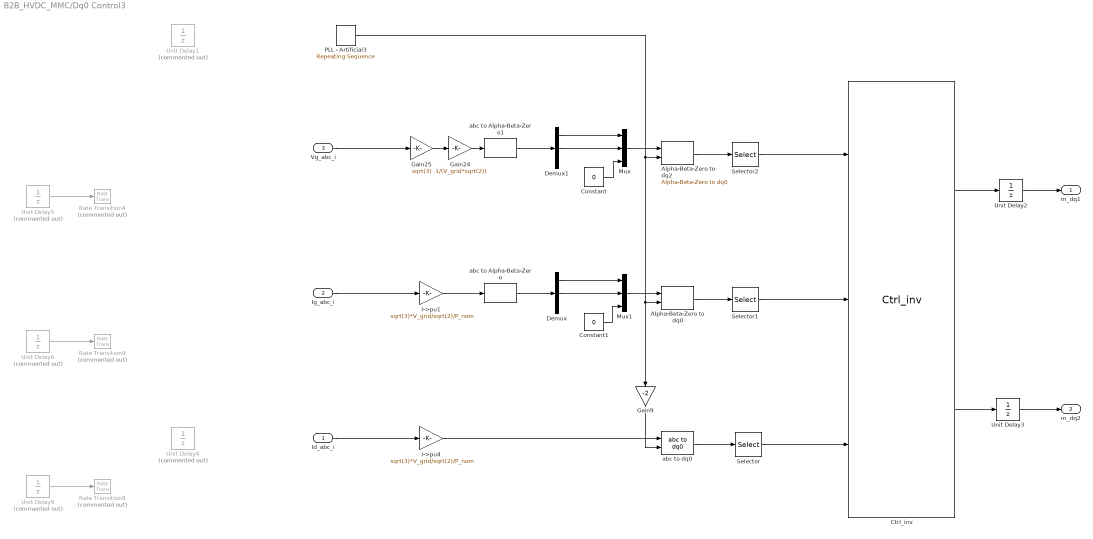
== system B2B_HVDC_MMC/Dq0 Control3 ==
  Id_abc_i : Inport
  Ig_abc_i : Inport  Port=2
  Vg_abc_i : Inport  Port=3
  Alpha-Beta-Zero to dq0 : spsAlphaBetaZerotodq0Lib/Alpha-Beta-Zero to dq0  Alignment=90 degrees behind phase A axis
  Alpha-Beta-Zero to dq2 : spsAlphaBetaZerotodq0Lib/Alpha-Beta-Zero to dq0  Alignment=90 degrees behind phase A axis
  Constant : Constant  Value=0
  Constant1 : Constant  Value=0
  Ctrl_inv : B2B_HVDC_MMC_Lib/Ctrl_inv  SystemSampleTime=-1  VariantActivationTime=update diagram  AllowFlexibleInterface=on  Latency=0  AutoFrameSizeCalculation=off
      settings: SourceProductName=BackToBack HVDC MMC Library
  Demux : Demux  Outputs=3
  Demux1 : Demux  Outputs=3
  Gain24 : Gain  Gain=1/(V_grid*sqrt(2))
  Gain25 : Gain  Gain=sqrt(3)
  Gain9 : Gain  Gain=-2
  I->pu1 : Gain  Gain=sqrt(3)*V_grid/sqrt(2)/P_nom  SaturateOnIntegerOverflow=on  OutDataTypeStr=Inherit: Same as input  ParamDataTypeStr=Inherit: Same as input
  I->pu4 : Gain  Gain=sqrt(3)*V_grid/sqrt(2)/P_nom  SaturateOnIntegerOverflow=on  OutDataTypeStr=Inherit: Same as input  ParamDataTypeStr=Inherit: Same as input
  Mux : Mux  Inputs=3
  Mux1 : Mux  Inputs=3
  PLL - Artificial3 : simulink/Sources/Repeating Sequence  rep_seq_t=[0 1/f]  rep_seq_y=[0 2*pi]
  Rate Transition4 : RateTransition  Commented=on  OutPortSampleTime=Ts_Control
  Rate Transition8 : RateTransition  Commented=on  OutPortSampleTime=Ts_Control
  Rate Transition9 : RateTransition  Commented=on  OutPortSampleTime=Ts_Control
  Selector : Selector  InputPortWidth=3  IndexOptions=Index vector (dialog)  Indices=[1 2]  OutputSizes=1
  Selector1 : Selector  InputPortWidth=3  IndexOptions=Index vector (dialog)  Indices=[1 2]  OutputSizes=1
  Selector2 : Selector  InputPortWidth=3  IndexOptions=Index vector (dialog)  Indices=[1 2]  OutputSizes=1
  Unit Delay{1,4..6,9} (5 alike) : UnitDelay  Commented=on  SampleTime=Ts_Power  HasFrameUpgradeWarning=on
  Unit Delay2 : UnitDelay  SampleTime=Ts_Power  HasFrameUpgradeWarning=on
  Unit Delay3 : UnitDelay  SampleTime=Ts_Power  HasFrameUpgradeWarning=on
  abc to Alpha-Beta-Zero : spsabctoAlphaBetaZeroLib/abc to Alpha-Beta-Zero
  abc to Alpha-Beta-Zero1 : spsabctoAlphaBetaZeroLib/abc to Alpha-Beta-Zero
  abc to dq0 : spsabctodq0Lib/abc to dq0  Alignment=90 degrees behind phase A axis
  m_dq1 : Outport  VectorParamsAs1DForOutWhenUnconnected=off
  m_dq2 : Outport  Port=2  VectorParamsAs1DForOutWhenUnconnected=off
  wires:
  Constant/1 -> Mux/3
  Demux/2 -> Mux1/2
  Demux/1 -> Mux1/1
  Mux1/1 -> Alpha-Beta-Zero to dq0/1
  Demux1/1 -> Mux/1
  Demux1/2 -> Mux/2
  Mux/1 -> Alpha-Beta-Zero to dq2/1
  abc to Alpha-Beta-Zero1/1 -> Demux1/1
  Alpha-Beta-Zero to dq2/1 -> Selector2/1
  Gain24/1 -> abc to Alpha-Beta-Zero1/1
  abc to Alpha-Beta-Zero/1 -> Demux/1
  I->pu1/1 -> abc to Alpha-Beta-Zero/1
  Gain25/1 -> Gain24/1
  Constant1/1 -> Mux1/3
  PLL - Artificial3/1 -> Alpha-Beta-Zero to dq2/2, Alpha-Beta-Zero to dq0/2, Gain9/1
  Gain9/1 -> abc to dq0/2
  I->pu4/1 -> abc to dq0/1
  Selector2/1 -> Ctrl_inv/1
  Selector1/1 -> Ctrl_inv/2
  Selector/1 -> Ctrl_inv/3
  Ctrl_inv/1 -> Unit Delay2/1
  Ctrl_inv/2 -> Unit Delay3/1
  Alpha-Beta-Zero to dq0/1 -> Selector1/1
  abc to dq0/1 -> Selector/1
  Unit Delay9/1 -> Rate Transition8/1
  Unit Delay6/1 -> Rate Transition9/1
  Unit Delay5/1 -> Rate Transition4/1
  Vg_abc_i/1 -> Gain25/1
  Ig_abc_i/1 -> I->pu1/1
  Id_abc_i/1 -> I->pu4/1
  Unit Delay2/1 -> m_dq1/1
  Unit Delay3/1 -> m_dq2/1

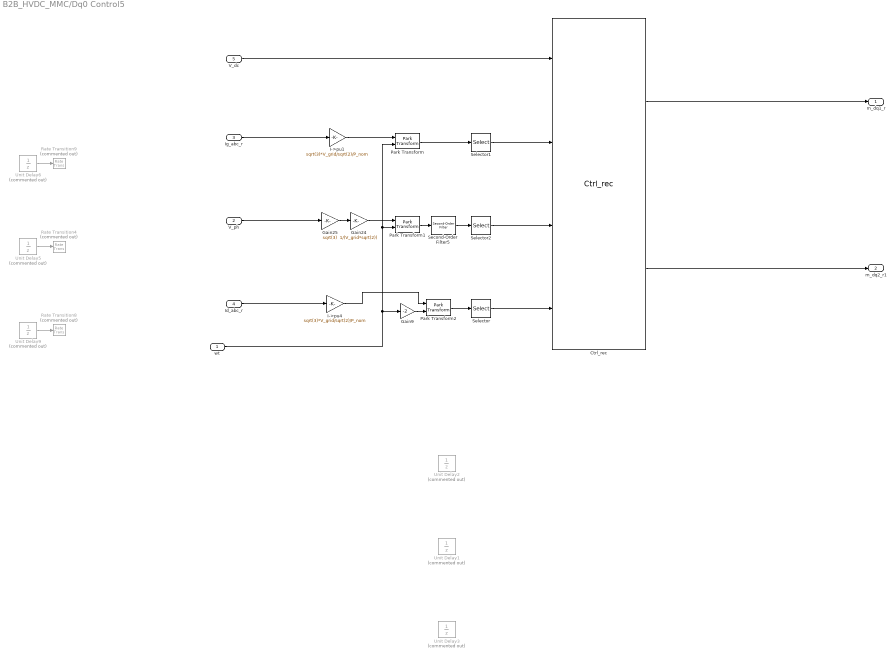
== system B2B_HVDC_MMC/Dq0 Control5 ==
  wt : Inport
  V_ph : Inport  Port=2
  Ig_abc_r : Inport  Port=3
  Id_abc_r : Inport  Port=4
  V_dc : Inport  Port=5
  Ctrl_rec : B2B_HVDC_MMC_Lib/Ctrl_rec  SystemSampleTime=-1  VariantActivationTime=update diagram  AllowFlexibleInterface=on  Latency=0  AutoFrameSizeCalculation=off
      settings: SourceProductName=BackToBack HVDC MMC Library
  Gain24 : Gain  Gain=1/(V_grid*sqrt(2))
  Gain25 : Gain  Gain=sqrt(3)
  Gain9 : Gain  Gain=-2
  I->pu1 : Gain  Gain=sqrt(3)*V_grid/sqrt(2)/P_nom  SaturateOnIntegerOverflow=on  OutDataTypeStr=Inherit: Same as input  ParamDataTypeStr=Inherit: Same as input
  I->pu4 : Gain  Gain=sqrt(3)*V_grid/sqrt(2)/P_nom  SaturateOnIntegerOverflow=on  OutDataTypeStr=Inherit: Same as input  ParamDataTypeStr=Inherit: Same as input
  Park Transform : eeTransforms/Park Transform  AxisAlignment=Q-axis  PowerInvariant=off
  Park Transform1 : eeTransforms/Park Transform  AxisAlignment=Q-axis  PowerInvariant=off
  Park Transform2 : eeTransforms/Park Transform  AxisAlignment=Q-axis  PowerInvariant=off
  Rate Transition4 : RateTransition  Commented=on  OutPortSampleTime=Ts_Control
  Rate Transition8 : RateTransition  Commented=on  OutPortSampleTime=Ts_Control
  Rate Transition9 : RateTransition  Commented=on  OutPortSampleTime=Ts_Control
  Second-Order Filter5 : spsSecondOrderFilterLib/Second-Order Filter  FilterType=Lowpass  Fo=Fn_filter  Zeta=Zeta_filter  Ts=Ts_Control  Initialize=off  Vac_Init="[0,  0,  60]"  Vdc_Init=0  PlotResponse=off  FreqRange=[0, 500, 1]
  Selector : Selector  InputPortWidth=3  IndexOptions=Index vector (dialog)  Indices=[1 2]  OutputSizes=1
  Selector1 : Selector  InputPortWidth=3  IndexOptions=Index vector (dialog)  Indices=[1 2]  OutputSizes=1
  Selector2 : Selector  InputPortWidth=3  IndexOptions=Index vector (dialog)  Indices=[1 2]  OutputSizes=1
  Unit Delay{1..3,5..6,9} (6 alike) : UnitDelay  Commented=on  SampleTime=Ts_Power  HasFrameUpgradeWarning=on
  m_dq1_r : Outport
  m_dq2_r1 : Outport  Port=2
  wires:
  I->pu1/1 -> Park Transform/1
  Gain25/1 -> Gain24/1
  Second-Order Filter5/1 -> Selector2/1
  Park Transform1/1 -> Second-Order Filter5/1
  Gain24/1 -> Park Transform1/1
  wt/1 -> Gain9/1, Park Transform1/2, Park Transform/2
  Gain9/1 -> Park Transform2/2
  Park Transform2/1 -> Selector/1
  V_dc/1 -> Ctrl_rec/1
  Selector1/1 -> Ctrl_rec/2
  Selector2/1 -> Ctrl_rec/3
  Selector/1 -> Ctrl_rec/4
  Ctrl_rec/1 -> m_dq1_r/1
  Ctrl_rec/2 -> m_dq2_r1/1
  I->pu4/1 -> Park Transform2/1
  Unit Delay9/1 -> Rate Transition8/1
  Unit Delay6/1 -> Rate Transition9/1
  Unit Delay5/1 -> Rate Transition4/1
  Park Transform/1 -> Selector1/1
  V_ph/1 -> Gain25/1
  Ig_abc_r/1 -> I->pu1/1
  Id_abc_r/1 -> I->pu4/1

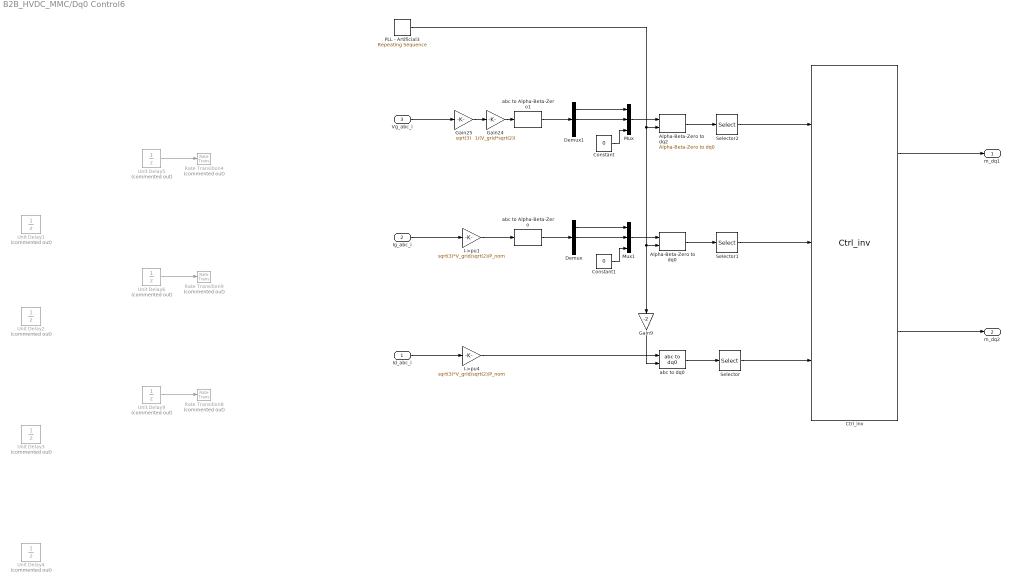
== system B2B_HVDC_MMC/Dq0 Control6 ==
  Id_abc_i : Inport
  Ig_abc_i : Inport  Port=2
  Vg_abc_i : Inport  Port=3
  Alpha-Beta-Zero to dq0 : spsAlphaBetaZerotodq0Lib/Alpha-Beta-Zero to dq0  Alignment=90 degrees behind phase A axis
  Alpha-Beta-Zero to dq2 : spsAlphaBetaZerotodq0Lib/Alpha-Beta-Zero to dq0  Alignment=90 degrees behind phase A axis
  Constant : Constant  Value=0
  Constant1 : Constant  Value=0
  Ctrl_inv : B2B_HVDC_MMC_Lib/Ctrl_inv  SystemSampleTime=-1  VariantActivationTime=update diagram  AllowFlexibleInterface=on  Latency=0  AutoFrameSizeCalculation=off
      settings: SourceProductName=BackToBack HVDC MMC Library
  Demux : Demux  Outputs=3
  Demux1 : Demux  Outputs=3
  Gain24 : Gain  Gain=1/(V_grid*sqrt(2))
  Gain25 : Gain  Gain=sqrt(3)
  Gain9 : Gain  Gain=-2
  I->pu1 : Gain  Gain=sqrt(3)*V_grid/sqrt(2)/P_nom  SaturateOnIntegerOverflow=on  OutDataTypeStr=Inherit: Same as input  ParamDataTypeStr=Inherit: Same as input
  I->pu4 : Gain  Gain=sqrt(3)*V_grid/sqrt(2)/P_nom  SaturateOnIntegerOverflow=on  OutDataTypeStr=Inherit: Same as input  ParamDataTypeStr=Inherit: Same as input
  Mux : Mux  Inputs=3
  Mux1 : Mux  Inputs=3
  PLL - Artificial3 : simulink/Sources/Repeating Sequence  rep_seq_t=[0 1/f]  rep_seq_y=[0 2*pi]
  Rate Transition4 : RateTransition  Commented=on  OutPortSampleTime=Ts_Control
  Rate Transition8 : RateTransition  Commented=on  OutPortSampleTime=Ts_Control
  Rate Transition9 : RateTransition  Commented=on  OutPortSampleTime=Ts_Control
  Selector : Selector  InputPortWidth=3  IndexOptions=Index vector (dialog)  Indices=[1 2]  OutputSizes=1
  Selector1 : Selector  InputPortWidth=3  IndexOptions=Index vector (dialog)  Indices=[1 2]  OutputSizes=1
  Selector2 : Selector  InputPortWidth=3  IndexOptions=Index vector (dialog)  Indices=[1 2]  OutputSizes=1
  Unit Delay{1..6,9} (7 alike) : UnitDelay  Commented=on  SampleTime=Ts_Power  HasFrameUpgradeWarning=on
  abc to Alpha-Beta-Zero : spsabctoAlphaBetaZeroLib/abc to Alpha-Beta-Zero
  abc to Alpha-Beta-Zero1 : spsabctoAlphaBetaZeroLib/abc to Alpha-Beta-Zero
  abc to dq0 : spsabctodq0Lib/abc to dq0  Alignment=90 degrees behind phase A axis
  m_dq1 : Outport  VectorParamsAs1DForOutWhenUnconnected=off
  m_dq2 : Outport  Port=2  VectorParamsAs1DForOutWhenUnconnected=off
  wires:
  Constant/1 -> Mux/3
  Demux/2 -> Mux1/2
  Demux/1 -> Mux1/1
  Mux1/1 -> Alpha-Beta-Zero to dq0/1
  Demux1/1 -> Mux/1
  Demux1/2 -> Mux/2
  Mux/1 -> Alpha-Beta-Zero to dq2/1
  abc to Alpha-Beta-Zero1/1 -> Demux1/1
  Alpha-Beta-Zero to dq2/1 -> Selector2/1
  Gain24/1 -> abc to Alpha-Beta-Zero1/1
  abc to Alpha-Beta-Zero/1 -> Demux/1
  I->pu1/1 -> abc to Alpha-Beta-Zero/1
  Gain25/1 -> Gain24/1
  Constant1/1 -> Mux1/3
  PLL - Artificial3/1 -> Alpha-Beta-Zero to dq2/2, Alpha-Beta-Zero to dq0/2, Gain9/1
  Gain9/1 -> abc to dq0/2
  I->pu4/1 -> abc to dq0/1
  Selector2/1 -> Ctrl_inv/1
  Selector1/1 -> Ctrl_inv/2
  Selector/1 -> Ctrl_inv/3
  Ctrl_inv/1 -> m_dq1/1
  Ctrl_inv/2 -> m_dq2/1
  Alpha-Beta-Zero to dq0/1 -> Selector1/1
  abc to dq0/1 -> Selector/1
  Unit Delay9/1 -> Rate Transition8/1
  Unit Delay6/1 -> Rate Transition9/1
  Unit Delay5/1 -> Rate Transition4/1
  Vg_abc_i/1 -> Gain25/1
  Ig_abc_i/1 -> I->pu1/1
  Id_abc_i/1 -> I->pu4/1

== system B2B_HVDC_MMC/Dq0 Control8 ==
  Id_DQN_i : Inport
  Ig_DQN_i : Inport  Port=2
  Vg_DQN_i : Inport  Port=3
  Ctrl_inv : B2B_HVDC_MMC_Lib/Ctrl_inv  SystemSampleTime=-1  VariantActivationTime=update diagram  AllowFlexibleInterface=on  Latency=0  AutoFrameSizeCalculation=off
      settings: SourceProductName=BackToBack HVDC MMC Library
  Gain1 : Gain  Gain=1/(V_grid*sqrt(2))
  Gain2 : Gain  Gain=sqrt(3)
  I->pu1 : Gain  Gain=sqrt(3)*V_grid/sqrt(2)/P_nom  SaturateOnIntegerOverflow=on  OutDataTypeStr=Inherit: Same as input  ParamDataTypeStr=Inherit: Same as input
  I->pu2 : Gain  Gain=sqrt(3)*V_grid/sqrt(2)/P_nom  SaturateOnIntegerOverflow=on  OutDataTypeStr=Inherit: Same as input  ParamDataTypeStr=Inherit: Same as input
  Selector1 : Selector  InputPortWidth=6*(N+1)  IndexOptions=Index vector (dialog)  Indices=[1*(N+1)+3 4*(N+1)+3]  OutputSizes=1
  Selector2 : Selector  InputPortWidth=6*(N+1)  IndexOptions=Index vector (dialog)  Indices=[2 3*(N+1)+2]  OutputSizes=1
  Selector3 : Selector  InputPortWidth=6*(N+1)  IndexOptions=Index vector (dialog)  Indices=[2 3*(N+1)+2]  OutputSizes=1
  Subsystem : Subsystem  Commented=on
  Unit Delay1 : UnitDelay  Commented=on  SampleTime=Ts_Power  HasFrameUpgradeWarning=on
  Unit Delay2 : UnitDelay  Commented=on  SampleTime=Ts_Power  HasFrameUpgradeWarning=on
  Unit Delay3 : UnitDelay  Commented=on  SampleTime=Ts_Power  HasFrameUpgradeWarning=on
  m_dq1 : Outport  VectorParamsAs1DForOutWhenUnconnected=off
  m_dq2 : Outport  Port=2  VectorParamsAs1DForOutWhenUnconnected=off
  wires:
  Gain1/1 -> Selector3/1
  Selector1/1 -> Ctrl_inv/3
  Gain2/1 -> Gain1/1
  I->pu2/1 -> Selector2/1
  I->pu1/1 -> Selector1/1
  Vg_DQN_i/1 -> Gain2/1
  Id_DQN_i/1 -> I->pu1/1
  Ig_DQN_i/1 -> I->pu2/1
  Selector3/1 -> Ctrl_inv/1
  Selector2/1 -> Ctrl_inv/2
  Ctrl_inv/1 -> m_dq1/1
  Ctrl_inv/2 -> m_dq2/1

== system B2B_HVDC_MMC/Dq0 Control9 ==
  wt : Inport
  V_ph : Inport  Port=2
  Ig_abc_r : Inport  Port=3
  Id_abc_r : Inport  Port=4
  V_dc : Inport  Port=5
  Ctrl_rec : B2B_HVDC_MMC_Lib/Ctrl_rec  SystemSampleTime=-1  VariantActivationTime=update diagram  Latency=0  AutoFrameSizeCalculation=off
      settings: SourceProductName=BackToBack HVDC MMC Library
  Gain24 : Gain  Gain=1/(V_grid*sqrt(2))
  Gain25 : Gain  Gain=sqrt(3)
  Gain9 : Gain  Gain=-2
  I->pu1 : Gain  Gain=sqrt(3)*V_grid/sqrt(2)/P_nom  SaturateOnIntegerOverflow=on  OutDataTypeStr=Inherit: Same as input  ParamDataTypeStr=Inherit: Same as input
  I->pu4 : Gain  Gain=sqrt(3)*V_grid/sqrt(2)/P_nom  SaturateOnIntegerOverflow=on  OutDataTypeStr=Inherit: Same as input  ParamDataTypeStr=Inherit: Same as input
  Park Transform : eeTransforms/Park Transform  AxisAlignment=Q-axis  PowerInvariant=off
  Park Transform1 : eeTransforms/Park Transform  AxisAlignment=Q-axis  PowerInvariant=off
  Park Transform2 : eeTransforms/Park Transform  AxisAlignment=Q-axis  PowerInvariant=off
  Rate Transition4 : RateTransition  Commented=on  OutPortSampleTime=Ts_Control
  Rate Transition8 : RateTransition  Commented=on  OutPortSampleTime=Ts_Control
  Rate Transition9 : RateTransition  Commented=on  OutPortSampleTime=Ts_Control
  Second-Order Filter5 : spsSecondOrderFilterLib/Second-Order Filter  FilterType=Lowpass  Fo=Fn_filter  Zeta=Zeta_filter  Ts=Ts_Control  Initialize=off  Vac_Init="[0,  0,  60]"  Vdc_Init=0  PlotResponse=off  FreqRange=[0, 500, 1]
  Selector : Selector  InputPortWidth=3  IndexOptions=Index vector (dialog)  Indices=[1 2]  OutputSizes=1
  Selector1 : Selector  InputPortWidth=3  IndexOptions=Index vector (dialog)  Indices=[1 2]  OutputSizes=1
  Selector2 : Selector  InputPortWidth=3  IndexOptions=Index vector (dialog)  Indices=[1 2]  OutputSizes=1
  Unit Delay{1..3,5..6,9} (6 alike) : UnitDelay  Commented=on  SampleTime=Ts_Power  HasFrameUpgradeWarning=on
  m_dq1_r : Outport
  m_dq2_r1 : Outport  Port=2
  wires:
  I->pu1/1 -> Park Transform/1
  Gain25/1 -> Gain24/1
  Second-Order Filter5/1 -> Selector2/1
  Park Transform1/1 -> Second-Order Filter5/1
  Gain24/1 -> Park Transform1/1
  wt/1 -> Gain9/1, Park Transform1/2, Park Transform/2
  Gain9/1 -> Park Transform2/2
  Park Transform2/1 -> Selector/1
  V_dc/1 -> Ctrl_rec/1
  Selector1/1 -> Ctrl_rec/2
  Selector2/1 -> Ctrl_rec/3
  Selector/1 -> Ctrl_rec/4
  Ctrl_rec/1 -> m_dq1_r/1
  Ctrl_rec/2 -> m_dq2_r1/1
  I->pu4/1 -> Park Transform2/1
  Unit Delay9/1 -> Rate Transition8/1
  Unit Delay6/1 -> Rate Transition9/1
  Unit Delay5/1 -> Rate Transition4/1
  Park Transform/1 -> Selector1/1
  V_ph/1 -> Gain25/1
  Ig_abc_r/1 -> I->pu1/1
  Id_abc_r/1 -> I->pu4/1

== system B2B_HVDC_MMC/Extra Sequences and functionality (Normally turned off) ==
  note: Iq controllers for converters
  note: Used for start-up simulation
  Enable Harmonic Filters : Step  Time=0  SampleTime=0
  Enable Reactive power setpoint regulation - (iq reference for inverter) : Step  Time=0.1  SampleTime=0  ZeroCross=off
  Energize Converters with startup current - Bypasses startup resistors : Step  Time=0.4  SampleTime=0
  Energize grid Harmonic Filter : Step  Time=0.1*0  SampleTime=0
  Grid Voltage stabilizer TURN ON - (iq reference for rectifier) : Step  Time=3  SampleTime=0
  tag scope: T_Energize=global, T_Harmonic1=global, T_iq_reg_i=global, T_iq_reg_r=global, T_startup=global
  wires:
  Energize grid Harmonic Filter/1 -> [T_Energize]
  Enable Reactive power setpoint regulation - (iq reference for inverter)/1 -> [T_iq_reg_i]
  Energize Converters with startup current - Bypasses startup resistors/1 -> [T_startup]
  Grid Voltage stabilizer TURN ON - (iq reference for rectifier)/1 -> [T_iq_reg_r]
  Enable Harmonic Filters/1 -> [T_Harmonic1]
